simulink model "Figure_3_2_TP_ReceptionFrequencePorteuse"  (R2020a)
settings: Solver=VariableStepAuto  StartTime=0.0  StopTime=10.0  RelTol=1e-3
model workspace (MAT data in the model file):
  K = Simulink.Parameter
  K.DataType = 'auto'
  K.Dimensions = [0 0]
libraries: dspsrcs4 x3, commdigbbndam3 x2, commchan3 x1, dsparch4 x1, commsink2 x1, commfilt2 x1, commrandsrc3 x1
settings Model: Creator=iba  LastModifiedBy=iba

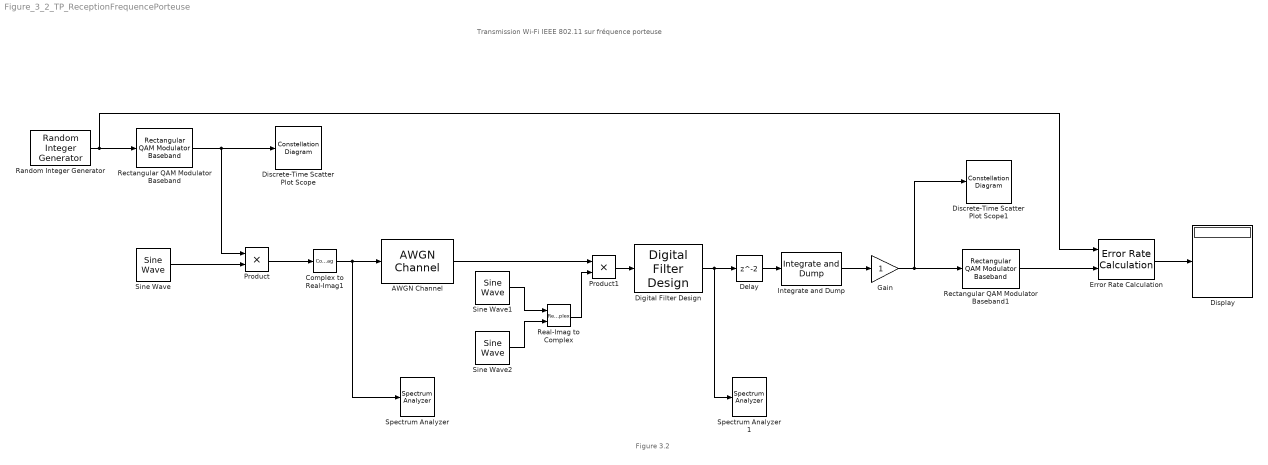
== system Figure_3_2_TP_ReceptionFrequencePorteuse ==
  note: Figure 3.2
  note: Transmission Wi-Fi IEEE 802.11 sur fréquence porteuse
  AWGN Channel : commchan3/AWGN Channel  InputProcessing=Columns as channels (frame based)  seed=67  noiseMode="Signal to noise ratio  (Eb/No)"  EbNodB=10  EsNodB=10  SNRdB=10  bitsPerSym=1  Ps=1  Tsym=1  variance=1
  Complex to Real-Imag1 : ComplexToRealImag  Output=Real
  Delay : Delay
  Digital Filter Design : dsparch4/Digital Filter Design  mwdsp_browser_bugfix_var=off
  Discrete-Time Scatter Plot Scope : ConstellationDiagram
  Discrete-Time Scatter Plot Scope1 : ConstellationDiagram
  Display : Display
  Error Rate Calculation : commsink2/Error Rate Calculation  N=1  st_delay=0  cp_mode=Entire frame  subframe=[]  PMode=Port  WsName=ErrorVec  RsMode2=off  stop=off  numErr=100  maxBits=1e6
  Gain : Gain
  Integrate and Dump : commfilt2/Integrate and Dump  obssamples=8  offsetsamples=0  nodump=off  roundingMode=Floor  overflowMode=off  outputDataTypeStr=Inherit: Same as accumulator  outputLastDataTypeStr=Inherit: Same as accumulator
  Product : Product
  Product1 : Product
  "Random Integer Generator " : commrandsrc3/Random Integer Generator  SetSize=8  SeedSource=Auto  Seed=0  SampleTime=1  SamplesPerFrame=1  OutputDataType=double  SimulateUsing=Interpreted execution
  Real-Imag to Complex : RealImagToComplex
  Rectangular QAM Modulator Baseband : commdigbbndam3/Rectangular QAM Modulator Baseband  M=64  InType=Integer  Enc=Gray  Mapping=[0:15]  PowType=Min. distance between symbols  MinDist=2  AvgPow=1  PeakPow=1  Ph=0  outDtype=double  outWordLen=16  outUDDataType=sfix(16)  outFracLenMode=Best precision  outFracLen=15  outDataTypeStr=double  outLastDataTypeStr=double
  Rectangular QAM Modulator Baseband1 : commdigbbndam3/Rectangular QAM Modulator Baseband  M=64  InType=Integer  Enc=Gray  Mapping=[0:15]  PowType=Min. distance between symbols  MinDist=2  AvgPow=1  PeakPow=1  Ph=0  outDtype=double  outWordLen=16  outUDDataType=sfix(16)  outFracLenMode=Best precision  outFracLen=15  outDataTypeStr=double  outLastDataTypeStr=double
  Sine Wave : dspsrcs4/Sine Wave  Amplitude=1  Frequency=100  Phase=0  SampleMode=Discrete  OutComplex=Real  CompMethod=Trigonometric fcn  TableSize=Speed  SampleTime=1/1000  SamplesPerFrame=1  ResetState=Restart at time zero  OutputFrames=off  dataType=double  wordLen=16  udDataType=sfix(16)  fracBitsMode=Best precision  numFracBits=15  OutDataTypeStr=double  LastOutDataTypeStr=double
  Sine Wave1 : dspsrcs4/Sine Wave  Amplitude=1  Frequency=100  Phase=0  SampleMode=Discrete  OutComplex=Real  CompMethod=Trigonometric fcn  TableSize=Speed  SampleTime=1/1000  SamplesPerFrame=1  ResetState=Restart at time zero  OutputFrames=off  dataType=double  wordLen=16  udDataType=sfix(16)  fracBitsMode=Best precision  numFracBits=15  OutDataTypeStr=double  LastOutDataTypeStr=double
  Sine Wave2 : dspsrcs4/Sine Wave  Amplitude=1  Frequency=100  Phase=0  SampleMode=Discrete  OutComplex=Real  CompMethod=Trigonometric fcn  TableSize=Speed  SampleTime=1/1000  SamplesPerFrame=1  ResetState=Restart at time zero  OutputFrames=off  dataType=double  wordLen=16  udDataType=sfix(16)  fracBitsMode=Best precision  numFracBits=15  OutDataTypeStr=double  LastOutDataTypeStr=double
  "Spectrum Analyzer " : SpectrumAnalyzer
  Spectrum Analyzer 1 : SpectrumAnalyzer
  wires:
  Product/1 -> Complex to Real-Imag1/1
  Complex to Real-Imag1/1 -> AWGN Channel/1, "Spectrum Analyzer "/1
  Rectangular QAM Modulator Baseband/1 -> Discrete-Time Scatter Plot Scope/1, Product/1
  Sine Wave/1 -> Product/2
  "Random Integer Generator "/1 -> Error Rate Calculation/1, Rectangular QAM Modulator Baseband/1
  Error Rate Calculation/1 -> Display/1
  Product1/1 -> Digital Filter Design/1
  Digital Filter Design/1 -> Spectrum Analyzer 1/1, Delay/1
  Sine Wave1/1 -> Real-Imag to Complex/1
  Sine Wave2/1 -> Real-Imag to Complex/2
  Real-Imag to Complex/1 -> Product1/2
  Delay/1 -> Integrate and Dump/1
  Integrate and Dump/1 -> Gain/1
  Gain/1 -> Discrete-Time Scatter Plot Scope1/1, Rectangular QAM Modulator Baseband1/1
  Rectangular QAM Modulator Baseband1/1 -> Error Rate Calculation/2
  AWGN Channel/1 -> Product1/1
